simulink model "Example_Composer"  (R2023b)
settings: Solver=VariableStepAuto  StartTime=0.0  StopTime=10.0  RelTol=1e-3
settings Model: Creator=22011083  LastModifiedBy=22011083

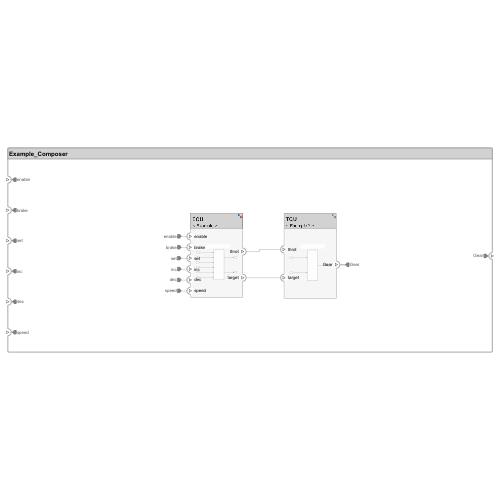
[thumbnail: Simulink's stored preview of the top-level diagram]
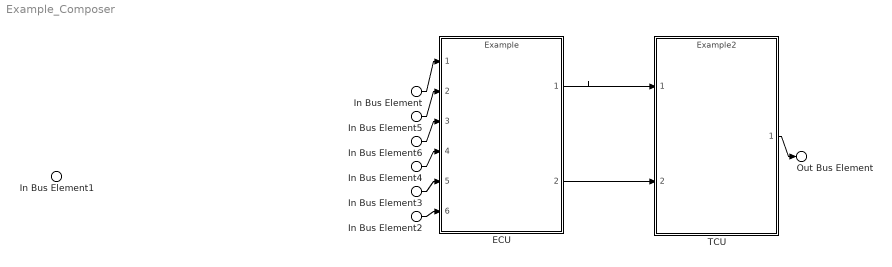
== system Example_Composer ==
  In Bus Element : Inport  PortName=enable
  In Bus Element1 : Inport  PortName=enable
  In Bus Element5 : Inport  Port=2  PortName=brake
  In Bus Element6 : Inport  Port=3  PortName=set
  In Bus Element4 : Inport  Port=4  PortName=inc
  In Bus Element3 : Inport  Port=5  PortName=dec
  In Bus Element2 : Inport  Port=6  PortName=speed
  ECU : ModelReference  ModelNameDialog=Example  SimulationMode=Normal  ModelReferenceVersion=6.9
      settings: PortSchema="{\"entries\":[{\"content\":{\"headerSize\":38,\"margin\":15,\"minimumSpacing\":25,\"sides\":[{\"content\":{\"connectorIds\":[\"In1\",\"In2\",\"In3\",\"In4\",\"In5\",\"In6\"]},\"type\":\"ConnectorPlacement.EquallySpacedRectSide\",\"uuid\":\"63d6e04c-e2bc-4f59-9952-e4bd1bc4b193\"},{\"content\":{\"connectorIds\":[\"Out1\",\"Out2\"],\"side\":\"RIGHT\"},\"type\":\"ConnectorPlacement.EquallySpacedRectSide\",\"uuid\":\"1ffa2562-6bc6-4ce4-b0e4-a17f0dd85330\"},{\"content\":{\"side\":\"TOP\"},\"type\":\"ConnectorPlacement.EquallySpacedRectSide\",\"uuid\":\"15fb3d64-5b7b-4f72-8832-d1d2c52621dc\"}]},\"type\":\"ConnectorPlacement.EquallySpacedConnector\",\"uuid\":\"c16ccf23-1ca1-40e4-bd3b-17a626dfb265\"}],\"packageUris\":[\"http://schema.mathworks.com/mf0/Connector/R2020b\"],\"version\":\"1.0\"}"
  TCU : ModelReference  ModelNameDialog=Example2  SimulationMode=Normal  ModelReferenceVersion=6.10
      settings: PortSchema="{\"entries\":[{\"content\":{\"headerSize\":38,\"margin\":15,\"minimumSpacing\":25,\"sides\":[{\"content\":{\"connectorIds\":[\"In1\",\"In2\"]},\"type\":\"ConnectorPlacement.EquallySpacedRectSide\",\"uuid\":\"63d6e04c-e2bc-4f59-9952-e4bd1bc4b193\"},{\"content\":{\"connectorIds\":[\"Out1\"],\"side\":\"RIGHT\"},\"type\":\"ConnectorPlacement.EquallySpacedRectSide\",\"uuid\":\"1ffa2562-6bc6-4ce4-b0e4-a17f0dd85330\"},{\"content\":{\"side\":\"TOP\"},\"type\":\"ConnectorPlacement.EquallySpacedRectSide\",\"uuid\":\"15fb3d64-5b7b-4f72-8832-d1d2c52621dc\"}]},\"type\":\"ConnectorPlacement.EquallySpacedConnector\",\"uuid\":\"c16ccf23-1ca1-40e4-bd3b-17a626dfb265\"}],\"packageUris\":[\"http://schema.mathworks.com/mf0/Connector/R2020b\"],\"version\":\"1.0\"}"
  Out Bus Element : Outport  PortName=Gear
  wires:
  In Bus Element/1 -> ECU/1
  In Bus Element5/1 -> ECU/2
  In Bus Element6/1 -> ECU/3
  In Bus Element4/1 -> ECU/4
  In Bus Element3/1 -> ECU/5
  In Bus Element2/1 -> ECU/6
  ECU/1 -> TCU/1
  ECU/2 -> TCU/2
  TCU/1 -> Out Bus Element/1
